simulink model "SmoothModelTFPade"  (R2020a)
settings: Solver=FixedStepAuto  StartTime=0  StopTime=10.67  FixedStep=0.01  RelTol=1e-3
undefined symbols (not defined in the file): K_D, K_P
libraries: cstblocks x1
settings Model: Creator=Brock  LastModifiedBy=Brock

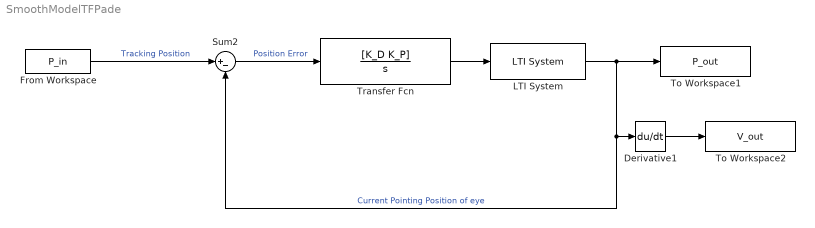
== system SmoothModelTFPade ==
  Derivative1 : Derivative
  From Workspace : FromWorkspace  VariableName=P_in
  LTI System : cstblocks/LTI System  sys=delayPade  IC=[]
  Sum2 : Sum  Inputs=|+-
  To Workspace1 : ToWorkspace  VariableName=P_out  SampleTime=-1
  To Workspace2 : ToWorkspace  VariableName=V_out  SampleTime=-1
  Transfer Fcn : TransferFcn  Numerator=[K_D K_P]  Denominator=[1 0]
  wires:
  LTI System/1 -> To Workspace1/1, Derivative1/1, Sum2/2  "Current Pointing Position of eye"
  From Workspace/1 -> Sum2/1  "Tracking Position"
  Derivative1/1 -> To Workspace2/1
  Sum2/1 -> Transfer Fcn/1  "Position Error"
  Transfer Fcn/1 -> LTI System/1
